simulink model "untitled"  (R2022b)
settings: Solver=FixedStepAuto  StartTime=0.0  StopTime=inf  FixedStep=0.3  RelTol=1e-3
libraries: robotmobilelib x2, rllib x1
settings Model: Creator=seif  LastModifiedBy=seif

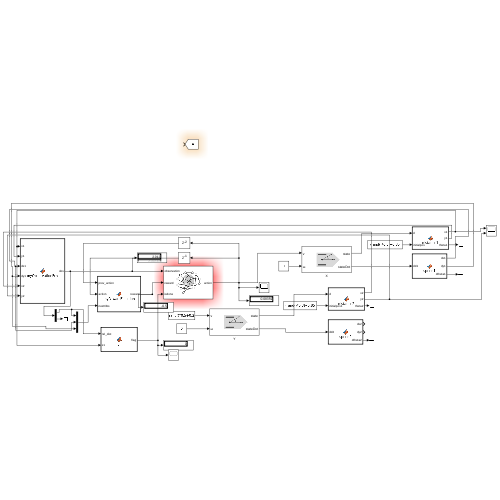
[thumbnail: Simulink's stored preview of the top-level diagram]
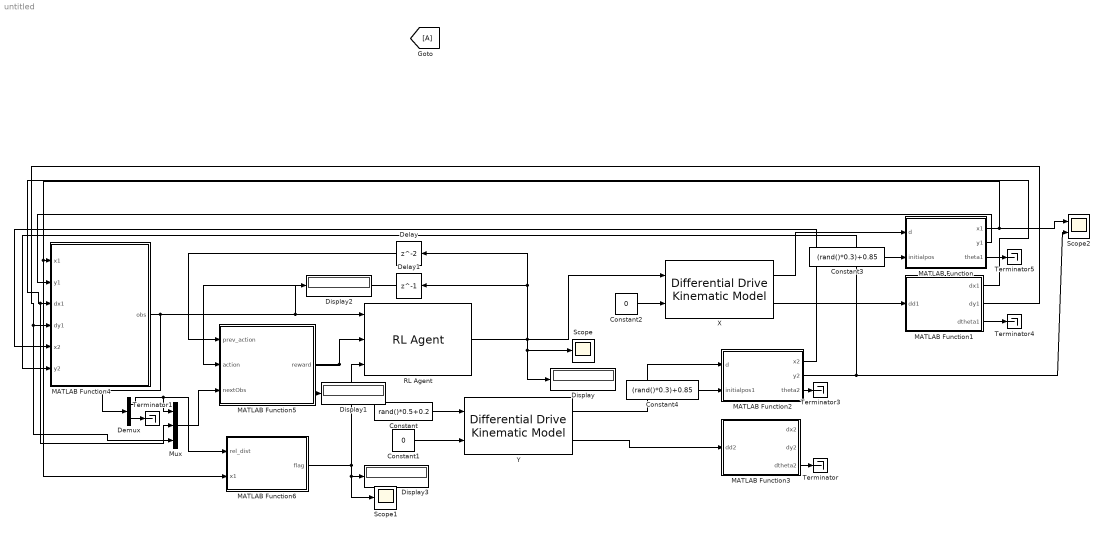
== system untitled ==
  Constant : Constant  Value=rand()*0.5+0.2
  Constant1 : Constant  Value=0
  Constant2 : Constant  Value=0
  Constant3 : Constant  Value=(rand()*0.3)+0.85
  Constant4 : Constant  Value=(rand()*0.3)+0.85
  Delay : Delay
  Delay1 : Delay  DelayLength=1
  Demux : Demux  Outputs=2
  Display{,1..3} (4 alike) : Display
  Goto : Goto
  MATLAB Function : MATLAB Function  TreatAsAtomicUnit=on
      settings: MinAlgLoopOccurrences=on
  MATLAB Function1 : MATLAB Function  TreatAsAtomicUnit=on
  MATLAB Function2 : MATLAB Function  TreatAsAtomicUnit=on
      settings: MinAlgLoopOccurrences=on
  MATLAB Function3 : MATLAB Function  TreatAsAtomicUnit=on
  MATLAB Function4 : MATLAB Function  TreatAsAtomicUnit=on
  MATLAB Function5 : MATLAB Function  TreatAsAtomicUnit=on
  MATLAB Function6 : MATLAB Function  TreatAsAtomicUnit=on
  Mux : Mux  Inputs=3
  RL Agent : rllib/RL Agent  Agent=agent1  ExternalActionAsInput=off  ProvideLastAction=off  ProvideCumRwd=off  TreatAsDirectFeedthrough=on  UseStrictObservationDataTypes=off
  Scope : Scope
  Scope1 : Scope
  Scope2 : Scope  NumInputPorts=2
  Terminator{,1,3..5} (5 alike) : Terminator
  X : robotmobilelib/Differential Drive Kinematic Model  VehicleInputs=Vehicle Speed & Heading Angular Velocity  WheelRadius=0.05  WheelSpeedRange=[-inf inf]  TrackWidth=0.2  InitialState=[0; 0; 0]  SimulateUsing=Interpreted execution
  Y : robotmobilelib/Differential Drive Kinematic Model  VehicleInputs=Vehicle Speed & Heading Angular Velocity  WheelRadius=0.05  WheelSpeedRange=[-inf inf]  TrackWidth=0.2  InitialState=[0; 0; 0]  SimulateUsing=Interpreted execution
  wires:
  X/1 -> MATLAB Function/1(d)
  X/2 -> MATLAB Function1/1(dd1)
  Y/1 -> MATLAB Function2/1(d)
  Y/2 -> MATLAB Function3/1(dd2)
  MATLAB Function4/1(obs) -> Demux/1, Display2/1, RL Agent/1
  MATLAB Function5/1(reward) -> RL Agent/2, Display1/1
  RL Agent/1 -> Display/1, Scope/1, Delay/1, Delay1/1, X/1
  Constant/1 -> Y/1
  Constant1/1 -> Y/2
  MATLAB Function3/3(dtheta2) -> Terminator/1
  Constant2/1 -> X/2
  Delay/1 -> MATLAB Function5/1(prev_action)
  Delay1/1 -> MATLAB Function5/2(action)
  Demux/2 -> Terminator1/1
  Mux/1 -> MATLAB Function5/3(nextObs)
  MATLAB Function2/3(theta2) -> Terminator3/1
  MATLAB Function1/3(dtheta1) -> Terminator4/1
  MATLAB Function/3(theta1) -> Terminator5/1
  MATLAB Function6/1(flag) -> RL Agent/3, Scope1/1, Display3/1
  Demux/1 -> MATLAB Function6/1(rel_dist), Mux/1
  MATLAB Function2/2(y2) -> MATLAB Function4/6(y2), Scope2/2
  MATLAB Function2/1(x2) -> MATLAB Function4/5(x2)
  MATLAB Function1/2(dy1) -> Mux/3, MATLAB Function4/4(dy1)
  MATLAB Function1/1(dx1) -> Mux/2, MATLAB Function4/3(dx1)
  MATLAB Function/1(x1) -> MATLAB Function6/2(x1), MATLAB Function4/1(x1), Scope2/1
  MATLAB Function/2(y1) -> MATLAB Function4/2(y1)
  Constant4/1 -> MATLAB Function2/2(initialpos1)
  Constant3/1 -> MATLAB Function/2(initialpos)

== matlab function untitled/MATLAB Function1 ==
  data: dd1 input; dx1 output; dy1 output; dtheta1 output
function [dx1, dy1, dtheta1] = speed1(dd1)
  % Perform some calculations on the input u to compute x, y, and theta
  dx1 = dd1(1);
  dy1 = dd1(2);
  dtheta1 = dd1(3);
  
  % Print the output values using sprintf
%   disp(['dx1 = ', sprintf('%f', dx1)]);
%   disp(['dy1 = ', sprintf('%f', dy1)]);
%   disp(['dtheta1 = ', sprintf('%f', dtheta1)]);
end

== matlab function untitled/MATLAB Function ==
  data: x1 output; y1 output; d input; theta1 output; initialpos input
function [x1, y1, theta1] = distance1(d,initialpos)
  % Perform some calculations on the input u to compute x, y, and theta
  
  
  x1 = d(1)-initialpos;
  y1 = 0;
  theta1 = d(3);
  
  % Print the output values using sprintf
%   disp(['x1 = ', sprintf('%f', x1)]);
%   disp(['y1 = ', sprintf('%f', y1)]);
%   disp(['theta1 = ', sprintf('%f', theta1)]);
  disp(['init = ', sprintf('%f', initialpos)]);
end

%((rand()*0.3)+0.85)

== matlab function untitled/MATLAB Function2 ==
  data: x2 output; y2 output; d input; theta2 output; initialpos1 input
function [x2, y2, theta2] = distance2(d,initialpos1)
  % Perform some calculations on the input u to compute x, y, and theta
%   rng('shuffle')
%   persistent initialpos1;
%   if isempty(initialpos1)
%     initialpos1 = ((rand()*0.3)+0.85);
%   end
  
  x2 = 0;
  y2 = d(1)-initialpos1;
  theta2 = d(3);

  
  % Print the output values using sprintf
%   disp(['x2 = ', sprintf('%f', x2)]);
%   disp(['y2 = ', sprintf('%f', y2)]);
%   disp(['theta2 = ', sprintf('%f', theta2)]);
    disp(['init2= ', sprintf('%f', initialpos1)])
end

== matlab function untitled/MATLAB Function3 ==
  data: dd2 input; dx2 output; dy2 output; dtheta2 output
function [dx2, dy2, dtheta2] = speed2(dd2)
  % Perform some calculations on the input u to compute x, y, and theta
  dx2 = dd2(1);
  dy2 = dd2(2);
  dtheta2 = dd2(3);
  
  % Print the output values using sprintf
%   disp(['dx2 = ', sprintf('%f', dx2)]);
%   disp(['dy2 = ', sprintf('%f', dy2)]);
%   disp(['dtheta2 = ', sprintf('%f', dtheta2)]);
end

== matlab function untitled/MATLAB Function4 ==
  data: x1 input; obs output; y1 input; dx1 input; dy1 input; x2 input; y2 input
function obs = myObservationFcn(x1, y1, dx1, dy1, x2, y2)
    % Calculate the relative distance between the two turtlebots
    rel_distance = sqrt((x1 - x2)^2 + (y1 - y2)^2);
    
    % Calculate the speeds of the two turtlebots
    speed1 = sqrt(dx1^2 + dy1^2);
%     speed2 = sqrt(dx2^2 + dy2^2);
    
    % Define the observation vector as [relative distance, speed1, speed2]
    obs = [rel_distance, speed1];
end

== matlab function untitled/MATLAB Function5 ==
  data: prev_action input; action input; reward output; nextObs input
function reward = myRewardFunction(prev_action, action, nextObs)

% Get the variables from nextObs
rel_dist = nextObs(1);
dx1 = nextObs(2);
dy1 = nextObs(3);


% Initialize the reward to zero
reward = 0;

% Penalize if turtlebot stops for more than 0.3 seconds
if abs(dx1) < 0.01 && abs(dy1) < 0.01 
    reward = reward - 1;
end

% Penalize if turtlebot is moving with low speed
if abs(dx1) < 0.1 && abs(dy1) < 0.1 
    reward = reward - 0.5;
end

% penalize collisions
if rel_dist < 0.3
    reward = reward - 50;

% penalize sudden changes in action   
diff = action - prev_action;
reward = reward - 0.1*norm(diff,1);


% Give reward if turtlebot passes a certain point
% if x1 > 5 && y1 > 5
%     reward = reward + 1;
% end

end

== matlab function untitled/MATLAB Function6 ==
  data: rel_dist input; flag output; x1 input
function flag = fcn(rel_dist,x1)

flag = rel_dist<0.3 || x1 >1.3;
    
end
